simulink model "thermal_IGBT_Loss"  (R2024b)
settings: Solver=VariableStepAuto  StartTime=0.0  StopTime=10  RelTol=1e-3
values from neighbouring files (symbols this model uses):
  alpha_AS_dB_km = 0.40    (= 0.4)    [Inverter_new.m]    (also in init_pv_inverter.m = 0.26)
  alpha_S_dB_km = 0.20    (= 0.2)    [Inverter_new.m]    (also in init_pv_inverter.m = 0.24)
  f_sw = 2000    [blindval.m]    (also in init_pv_inverter.m)
  Pload = 2000    [blindval.m]    (also in init_pv_inverter.m)
  Rinterface_h = 0.02    [blindval.m]    (also in init_pv_inverter.m)
  Ron_IGBT = 1e-3    (= 0.001)    [blindval.m]    (also in init_pv_inverter.m)
  RTI = 90    [init_pv_inverter.m]
  T_ambient_fibre = Ta_K    (= 298.15)    [init_pv_inverter.m]
  Ta = test_cases(k,2)    [blindval.m]    (also in init_pv_inverter.m = 25)
  tf_IGBT = 63e-9    (= 6.3e-08)    [degradation_states.m]    (also in degradations_states_new.m; generate_degradation.m; init_pv_inverter.m; run_degradation.m)
  tr_IGBT = 11e-9    (= 1.1e-08)    [degradation_states.m]    (also in degradations_states_new.m; generate_degradation.m; init_pv_inverter.m; run_degradation.m)
  Ts_pwm = 5e-5    (= 5e-05)    [init_pv_inverter.m]
  Vdc = test_cases(k,3)    [blindval.m]    (also in init_pv_inverter.m = 600)
  Vf_IGBT = 0.8    [blindval.m]    (also in init_pv_inverter.m)
  x_fibre = 0:dx:L_fibre    [init_pv_inverter.m]
  x_fibre_km = x_fibre / 1000    [init_pv_inverter.m]
  x_inv_end = 7    [init_pv_inverter.m]
  x_inv_start = 5    [init_pv_inverter.m]
libraries: nesl_utility x13, ee_lib x8, fl_lib x6, simulink x6, eePwmGeneratorTwoLevel x1
settings Model: Creator=tf  LastModifiedBy=tf

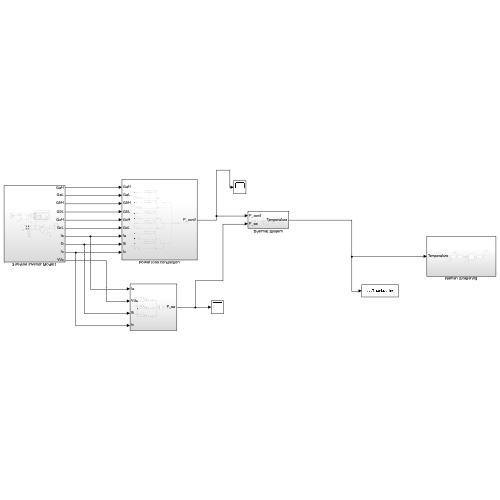
[thumbnail: Simulink's stored preview of the top-level diagram]
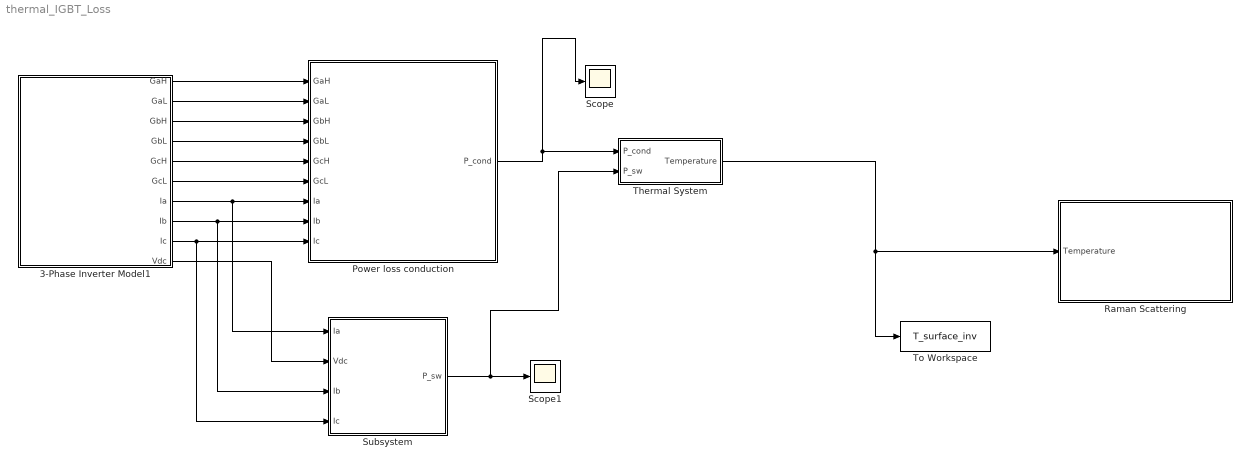
== system thermal_IGBT_Loss ==
  3-Phase Inverter Model1 : Subsystem
  Power loss conduction : Subsystem
  Raman Scattering : Subsystem
  Scope : Scope
  Scope1 : Scope
  Subsystem : Subsystem
  Thermal System : Subsystem
  To Workspace : ToWorkspace  VariableName=T_surface_inv  SaveFormat=Timeseries  SampleTime=0.01
  wires:
  Thermal System/1(Temperature) -> To Workspace/1, Raman Scattering/1(Temperature)
  3-Phase Inverter Model1/3(GbH) -> Power loss conduction/3(GbH)
  3-Phase Inverter Model1/7(Ia) -> Subsystem/1(Ia), Power loss conduction/7(Ia)
  3-Phase Inverter Model1/9(Ic) -> Subsystem/4(Ic), Power loss conduction/9(Ic)
  3-Phase Inverter Model1/2(GaL) -> Power loss conduction/2(GaL)
  3-Phase Inverter Model1/1(GaH) -> Power loss conduction/1(GaH)
  3-Phase Inverter Model1/5(GcH) -> Power loss conduction/5(GcH)
  3-Phase Inverter Model1/4(GbL) -> Power loss conduction/4(GbL)
  3-Phase Inverter Model1/6(GcL) -> Power loss conduction/6(GcL)
  3-Phase Inverter Model1/8(Ib) -> Subsystem/3(Ib), Power loss conduction/8(Ib)
  Power loss conduction/1(P_cond) -> Thermal System/1(P_cond), Scope/1
  3-Phase Inverter Model1/10(Vdc) -> Subsystem/2(Vdc)
  Subsystem/1(P_sw) -> Thermal System/2(P_sw), Scope1/1

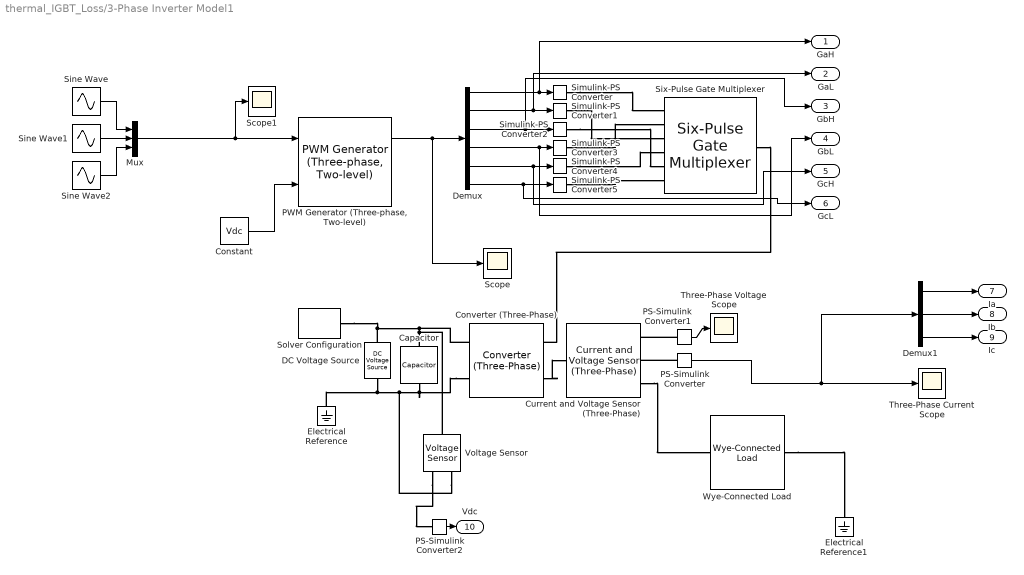
== system thermal_IGBT_Loss/3-Phase Inverter Model1 ==
  Capacitor : ee_lib/Passive/Capacitor  cap_option=ee.enum.passive.capacitor.capOption.const  c=1e-6 F  Cvec=[1e-05, 1e-06] F  Vvec=[0, 10] V  CV_table_symmetry=ee.enum.passive.capacitor.tableSymmetry.yes  f_vec=[1, 10] kHz  DFext_vec=[.8, 1.2]  enable_C_tol=ee.enum.toleranceApplication.none  averaging_period=0 s  C_tol=5  tol_distribution=ee.enum.toleranceDistribution.uniform  nSigma=4  r=0 Ohm  g=0 1/Ohm  enable_operating_limits=ee.enum.enable.no  operating_limit_action=ee.enum.passive.reportOpLim.warn  max_working_voltage_range=[-25, 25] V  power_rating=1 W  maxTemperature=85 degC  thermalEnable=false  thermalMass=1 J/K  fault_action=simscape.enum.assert.action.none  t_fault=1 s  i_specify=off  i_priority=None  i=0 A  i_nominal_specify=off  i_nominal_value=1  i_nominal_unit=A  v_specify=off  v_priority=High  v=600 V  v_nominal_specify=off  v_nominal_value=1  v_nominal_unit=V  vc_specify=on  vc_priority=High  vc=Vdc V  vc_nominal_specify=off  vc_nominal_value=1  vc_nominal_unit=V  T_specify=off  T_priority=None  T=298.15 K  T_nominal_specify=off  T_nominal_value=1  T_nominal_unit=K
  Constant : Constant  Value=Vdc
  Converter (Three-Phase) : ee_lib/Semiconductors & Converters/Converters/Converter (Three-Phase)  port_option=ee.enum.threePhasePort.composite  fidelity_option=ee.enum.converters.fidelity.equivalent_pwm  device_type=ee.enum.converters.switchingdevice.ideal  showThermalPort=true  K=0  Vth=6 V  Vgt=1 V  Vgt_off=-1 V  Ih=1 A  Vf=0.8 V  Ron=0.001 Ohm  Rds=0.001 Ohm  Goff=1e-6 1/Ohm  Eon_scalar=22.86e-3 J  Eoff_scalar=17.14e-3 J  Eoff_natural_commutation=10e-3 J  Voff=300 V  Iout_scalar=600 A  onCurrentMeasDelay=0 s  useCurrentFromPreviousCycle=false  useVoltageFromPreviousCycle=false  diode_param=ee.enum.converters.protectiondiode.nodynamics  diode_Vf=0.8 V  diode_Ron=0.001 Ohm  diode_Goff=1e-5 1/Ohm  diode_C=50 nF  diode_iRM=-235 A  diode_iF=300 A  diode_idot=-50 A/us  diode_trr_param=ee.enum.converters.diodetrr.trr_factor  diode_trr_factor=3  diode_trr=15 us  diode_Qrr=1500 s*uA  diode_rec_loss_model=ee.enum.diode.reverseRecoveryModel.fixed  diode_ErecVal=0 J  diode_scaleWithIandV=false  diode_ErecMat=zeros(2, 3) J  diode_TjrecVec=[298.15, 398.15] K  diode_IfrecVec=[.1, 1, 10] A  diode_IrecVal=10 A  diode_VrecVal=10 V  diode_tFilter=1 / 1000 / 100 s  thermal_network_parameterization=ee.enum.thermalNetworkTopology.external  Rth=[.08, .5] K/W  Rth_Cauer=[.08, .1, .5] K/W  Rth_Foster=[.08, .14, .22, .16] K/W  thermal_mass_parameterization=ee.enum.thermalNetwork.timeconstant  thermal_mass=[.01, .5] J/K  thermal_mass_Cauer=[.01, .1, .5] J/K  thermal_mass_Foster=[.001, .005, .05, .5] J/K  thermal_time_constant=[.001, .2] s  thermal_time_constant_Cauer=[.001, .1, .2] s  thermal_time_constant_Foster=[7e-05, .0007, .01, .08] s  thermal_mass_initial_temperatures=[25, 25] degC  thermal_mass_initial_temperatures_Cauer=[25, 25, 25] degC  junction_thermal_mass=0.01 J/K  Tvec_initial_Foster=[25, 25, 25, 25] degC  snubber_type=ee.enum.converters.snubber.exclude  Cs=1e-7 F  Rs=0.1 Ohm  Vce_loss=[0, 150, 300] V
  Current and Voltage Sensor (Three-Phase) : ee_lib/Sensors & Transducers/Current and Voltage Sensor (Three-Phase)  vMeasurementType=ee.enum.vmeasurement.lg  outputUnit=ee.enum.unit.si  SRated=100e6 A*V  VRated=24e3 V  I_specify=off  I_priority=None  I=[0, 0, 0] A  I_nominal_specify=off  I_nominal_value=1  I_nominal_unit=A  V_specify=off  V_priority=None  V=[0, 0, 0] V  V_nominal_specify=off  V_nominal_value=1  V_nominal_unit=V
      settings: InternalSimscapePortConfiguration="{\"Bottom\":[],\"Left\":[{\"id\":\"N1\",\"label\":\"~1\",\"type\":\"foundation.electrical.three_phase\"}],\"Right\":[{\"id\":\"V_output\",\"label\":\"V\",\"type\":\"output\"},{\"id\":\"I_output\",\"label\":\"I\",\"type\":\"output\"},{\"id\":\"N2\",\"label\":\"~2\",\"type\":\"foundation.electrical.three_phase\"}],\"Top\":[]}"
  DC Voltage Source : ee_lib/Additional Components/SPICE Sources/DC Voltage Source  DC=Vdc V
  Demux : Demux  Outputs=6
  Demux1 : Demux  Outputs=3
  Electrical Reference : fl_lib/Electrical/Electrical Elements/Electrical Reference
  Electrical Reference1 : fl_lib/Electrical/Electrical Elements/Electrical Reference
  Mux : Mux  Inputs=3
  PS-Simulink Converter : nesl_utility/PS-Simulink Converter  PhysicalDomain=network_engine_domain  SubClassName=ps_output  LeftPortType=input  RightPortType=output  PseudoPeriodic=off  Frequencies=[]  VectorFormat=inherit  Unit=A  AffineConversion=off
  PS-Simulink Converter1 : nesl_utility/PS-Simulink Converter  PhysicalDomain=network_engine_domain  SubClassName=ps_output  LeftPortType=input  RightPortType=output  PseudoPeriodic=off  Frequencies=[]  VectorFormat=inherit  Unit=V  AffineConversion=off
  PS-Simulink Converter2 : nesl_utility/PS-Simulink Converter  PhysicalDomain=network_engine_domain  SubClassName=ps_output  LeftPortType=input  RightPortType=output  PseudoPeriodic=off  Frequencies=[]  VectorFormat=inherit  Unit=V  AffineConversion=off
  "PWM Generator (Three-phase, Two-level)" : eePwmGeneratorTwoLevel/PWM Generator (Three-phase, Two-level)  PWMMode=Continuous PWM (CPWM)  CPWMMode=SPWM: sinusoidal PWM  DPWMMode=60 DPWM: 60 degree discontinuous PWM  fsw=f_sw  Ts=Ts_pwm
  Scope : Scope
  Scope1 : Scope
  Simulink-PS Converter{,1..5} (6 alike) : nesl_utility/Simulink-PS Converter  PhysicalDomain=network_engine_domain  SubClassName=ps_input  LeftPortType=input  RightPortType=output  PseudoPeriodic=off  Frequencies=[]  NoiseDistribution=none  NoiseParameters=[]  Unit=1  AffineConversion=off  FilteringAndDerivatives=provide  SimscapeFilterOrder=1  InputFilterTimeConstant=0.001  UdotUserProvided=0
  Sine Wave : Sin  Amplitude=0.8  Frequency=50  SampleTime=0
  Sine Wave1 : Sin  Amplitude=0.8  Frequency=50  Phase=-2*pi/3  SampleTime=0
  Sine Wave2 : Sin  Amplitude=0.8  Frequency=50  Phase=2*pi/3  SampleTime=0
  Six-Pulse Gate Multiplexer : ee_lib/Semiconductors & Converters/Converters/Six-Pulse Gate Multiplexer  port_option=ee.enum.controlport.ps
  Solver Configuration : nesl_utility/Solver Configuration  PhysicalDomain=network_engine_domain  SubClassName=solver  LeftPortType=input  RightPortType=generic  Tones=[]  Harmonics=[]  SimulateNoise=off  Profile=off  UseLocalSampling=off  EnableSwitchedLinearOptims=on  FrequencyDomain=off  UseCCode=off  RelTol=0.001  AbsTol=0.001  MinStep=1e-09  ToWorkspace=off  RevertToSquareIcSolve=off  NumHomotopyIterations=100  PhasorMode=off  PhasorModeNumHarmonics=1  ConsistencySolver=NEWTON_XTOL_AFTER_FTOL  IndexReductionMethod=DerivativeReplacement  DoDC=off  ResidualTolerance=1e-09  ConsistencyTolSource=GLOBAL  ConsistencyAbsTol=0.001  ConsistencyRelTol=0.001  ConsistencyTolFactor=0.001  UseLocalSolver=off  LocalSolverChoice=NE_BACKWARD_EULER_ADVANCER  ResolveIndetEquations=on  FunctionEvalNumThread=1  LocalSolverSampleTime=0.001  DoFixedCost=off  MaxNonlinIter=3  MaxModeIter=2  ComputeImpulses=off  ImpulseIterations=2  LinearAlgebra=auto  LinearAlgebraNumThread=0  EquationFormulation=NE_TIME_EF  DelaysMemoryBudget=1024  AutomaticFiltering=on  FilteringTimeConstant=0.001  PartitionStorageMethod=AS_NEEDED  PartitionMemoryBudget=1024  PartitionMethod=ROBUST  MultibodyUseLocalSolver=off  MultibodyLocalSolverChoice=ODE1  MultibodyLocalSolverSampleTime=0.001
  Three-Phase Current Scope : Scope
  Three-Phase Voltage Scope : Scope
  Voltage Sensor : fl_lib/Electrical/Electrical Sensors/Voltage Sensor
  Wye-Connected Load : ee_lib/Passive/RLC Assemblies/Wye-Connected Load  port_option=ee.enum.threePhasePort.composite  parameterization=ee.enum.rlc.parameterization.ratedpower  component_structure=ee.enum.rlc.structure.SeriesRL  component_structure_PQ=ee.enum.rlc.structure.SeriesRLC  R=1 Ohm  L=1e-3 H  C=1e-6 F  VRated=Vload_rated V  FRated=f_out Hz  P=Pload W  Qpos=Qind A*V  Qneg=Qcap A*V  R_parasitic=1e-6 Ohm  G_parasitic=1e-6 1/Ohm  R_parasitic_PQ=1e-6 Ohm  G_parasitic_PQ=1e-6 1/Ohm  Vmag0=24e3 V  Vang0=0 deg  Freq0=60 Hz  IL_specify=off  IL_priority=High  IL=[0, 0, 0] A  IL_nominal_specify=off  IL_nominal_value=1  IL_nominal_unit=A  VC_specify=off  VC_priority=High  VC=[0, 0, 0] V  VC_nominal_specify=off  VC_nominal_value=1  VC_nominal_unit=V
  GaH : Outport
  GaL : Outport  Port=2
  GbH : Outport  Port=3
  GbL : Outport  Port=4
  GcH : Outport  Port=5
  GcL : Outport  Port=6
  Ia : Outport  Port=7
  Ib : Outport  Port=8
  Ic : Outport  Port=9
  Vdc : Outport  Port=10
  wires:
  "PWM Generator (Three-phase, Two-level)"/1 -> Demux/1, Scope/1
  PS-Simulink Converter/1 -> Demux1/1, Three-Phase Current Scope/1
  Constant/1 -> "PWM Generator (Three-phase, Two-level)"/2
  Sine Wave/1 -> Mux/1
  Mux/1 -> Scope1/1, "PWM Generator (Three-phase, Two-level)"/1
  Demux/5 -> GcH/1, Simulink-PS Converter4/1
  Sine Wave1/1 -> Mux/2
  Demux/6 -> GcL/1, Simulink-PS Converter5/1
  Demux/4 -> GbL/1, Simulink-PS Converter3/1
  Demux/1 -> GaH/1, Simulink-PS Converter/1
  Sine Wave2/1 -> Mux/3
  Demux/2 -> GaL/1, Simulink-PS Converter1/1
  PS-Simulink Converter1/1 -> Three-Phase Voltage Scope/1
  Demux/3 -> GbH/1, Simulink-PS Converter2/1
  Demux1/1 -> Ia/1
  Demux1/2 -> Ib/1
  Demux1/3 -> Ic/1
  PS-Simulink Converter2/1 -> Vdc/1
  connections:
  Converter (Three-Phase)/RConn2 -- DC Voltage Source/RConn1 -- Electrical Reference/LConn1 -- Voltage Sensor/RConn2 -- Capacitor/RConn1
  Converter (Three-Phase)/RConn1 -- Voltage Sensor/LConn1 -- Capacitor/LConn1 -- DC Voltage Source/LConn1 -- Solver Configuration/RConn1
  Converter (Three-Phase)/LConn2 -- Current and Voltage Sensor (Three-Phase)/LConn1
  Six-Pulse Gate Multiplexer/RConn1 -- Converter (Three-Phase)/LConn1
  Simulink-PS Converter/RConn1 -- Six-Pulse Gate Multiplexer/LConn1
  PS-Simulink Converter/LConn1 -- Current and Voltage Sensor (Three-Phase)/RConn2
  Current and Voltage Sensor (Three-Phase)/RConn3 -- Wye-Connected Load/LConn1
  Wye-Connected Load/RConn1 -- Electrical Reference1/LConn1
  PS-Simulink Converter1/LConn1 -- Current and Voltage Sensor (Three-Phase)/RConn1
  Simulink-PS Converter3/RConn1 -- Six-Pulse Gate Multiplexer/LConn2
  Simulink-PS Converter1/RConn1 -- Six-Pulse Gate Multiplexer/LConn3
  Simulink-PS Converter4/RConn1 -- Six-Pulse Gate Multiplexer/LConn4
  Simulink-PS Converter2/RConn1 -- Six-Pulse Gate Multiplexer/LConn5
  Simulink-PS Converter5/RConn1 -- Six-Pulse Gate Multiplexer/LConn6
  Voltage Sensor/RConn1 -- PS-Simulink Converter2/LConn1

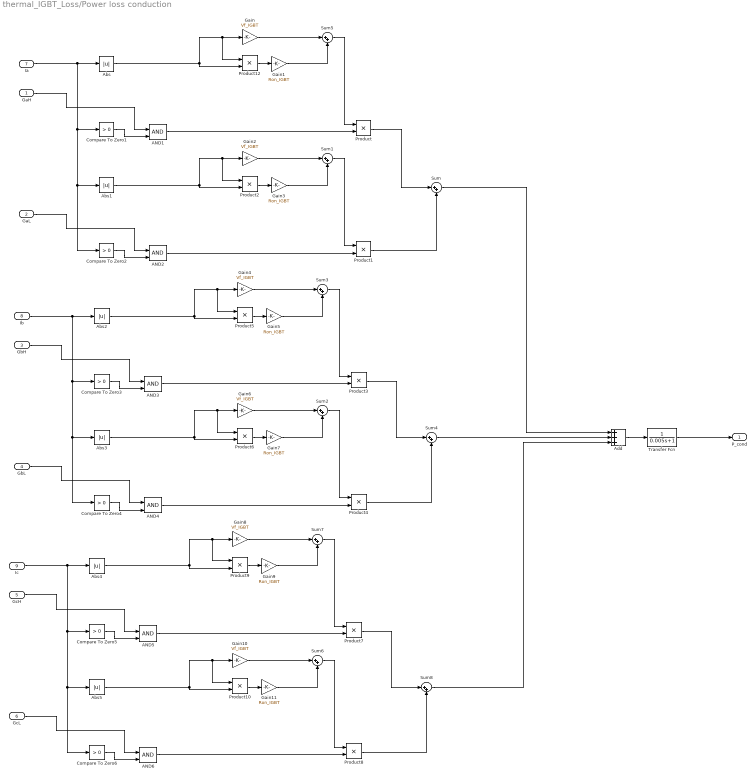
== system thermal_IGBT_Loss/Power loss conduction ==
  GaH : Inport
  GaL : Inport  Port=2
  GbH : Inport  Port=3
  GbL : Inport  Port=4
  GcH : Inport  Port=5
  GcL : Inport  Port=6
  Ia : Inport  Port=7
  Ib : Inport  Port=8
  Ic : Inport  Port=9
  AND{1..6} (6 alike) : Logic  IconShape=distinctive  AllPortsSameDT=off  OutDataTypeStr=boolean
  Abs{,1..5} (6 alike) : Abs  SaturateOnIntegerOverflow=off
  Add : Sum  Inputs=+++
  Compare To Zero{1..6} (6 alike) : simulink/Logic and Bit Operations/Compare To Zero  relop=>  OutDataTypeStr=boolean
  Gain{,2,4,6,8,10} (6 alike) : Gain  Gain=Vf_IGBT
  Gain{1,3,5,7,9,11} (6 alike) : Gain  Gain=Ron_IGBT
  Product{,1..10,12} (12 alike) : Product
  Sum{,1..8} (9 alike) : Sum  Inputs=|++
  Transfer Fcn : TransferFcn  Denominator=[0.005 1]
  P_cond : Outport
  wires:
  GaH/1 -> AND1/1
  Compare To Zero1/1 -> AND1/2
  Gain/1 -> Sum5/1
  Gain1/1 -> Sum5/2
  Product12/1 -> Gain1/1
  Abs/1 -> Product12/2, Product12/1, Gain/1
  AND1/1 -> Product/2
  Sum5/1 -> Product/1
  Product2/1 -> Gain3/1
  Ia/1 -> Compare To Zero2/1, Abs1/1, Compare To Zero1/1, Abs/1
  GaL/1 -> AND2/1
  Gain3/1 -> Sum1/2
  Abs1/1 -> Product2/2, Product2/1, Gain2/1
  AND2/1 -> Product1/2
  Gain2/1 -> Sum1/1
  Compare To Zero2/1 -> AND2/2
  Sum1/1 -> Product1/1
  AND4/1 -> Product4/2
  Gain5/1 -> Sum3/2
  Gain6/1 -> Sum2/1
  GbL/1 -> AND4/1
  Abs2/1 -> Product5/2, Product5/1, Gain4/1
  Abs3/1 -> Product6/2, Product6/1, Gain6/1
  Gain7/1 -> Sum2/2
  Product5/1 -> Gain5/1
  Compare To Zero4/1 -> AND4/2
  Product6/1 -> Gain7/1
  Sum2/1 -> Product4/1
  AND3/1 -> Product3/2
  GbH/1 -> AND3/1
  Gain4/1 -> Sum3/1
  Sum3/1 -> Product3/1
  Compare To Zero3/1 -> AND3/2
  Ib/1 -> Compare To Zero4/1, Abs3/1, Compare To Zero3/1, Abs2/1
  Product/1 -> Sum/1
  Product1/1 -> Sum/2
  Product3/1 -> Sum4/1
  Product4/1 -> Sum4/2
  Product10/1 -> Gain11/1
  Gain11/1 -> Sum6/2
  AND5/1 -> Product7/2
  Ic/1 -> Compare To Zero6/1, Abs5/1, Compare To Zero5/1, Abs4/1
  Abs5/1 -> Product10/2, Product10/1, Gain10/1
  Gain8/1 -> Sum7/1
  Product8/1 -> Sum8/2
  GcH/1 -> AND5/1
  Compare To Zero6/1 -> AND6/2
  Abs4/1 -> Product9/2, Product9/1, Gain8/1
  Sum6/1 -> Product8/1
  GcL/1 -> AND6/1
  Compare To Zero5/1 -> AND5/2
  Product9/1 -> Gain9/1
  Sum7/1 -> Product7/1
  Product7/1 -> Sum8/1
  AND6/1 -> Product8/2
  Gain9/1 -> Sum7/2
  Gain10/1 -> Sum6/1
  Sum/1 -> Add/1
  Sum4/1 -> Add/2
  Sum8/1 -> Add/3
  Add/1 -> Transfer Fcn/1
  Transfer Fcn/1 -> P_cond/1

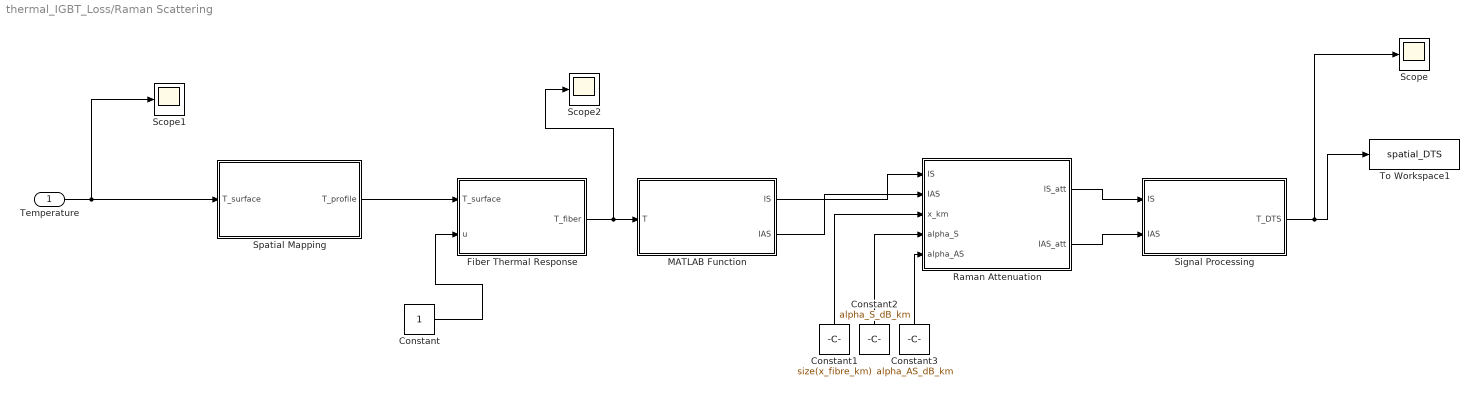
== system thermal_IGBT_Loss/Raman Scattering ==
  Temperature : Inport
  Constant : Constant
  Constant1 : Constant  Value=size(x_fibre_km)
  Constant2 : Constant  Value=alpha_S_dB_km
  Constant3 : Constant  Value=alpha_AS_dB_km
  Fiber Thermal Response : Subsystem
  MATLAB Function : MATLAB Function  TreatAsAtomicUnit=on
  Raman Attenuation : MATLAB Function  TreatAsAtomicUnit=on
  Scope : Scope
  Scope1 : Scope
  Scope2 : Scope
  Signal Processing : Subsystem
  Spatial Mapping : Subsystem
  To Workspace1 : ToWorkspace  VariableName=spatial_DTS  SaveFormat=Timeseries  SampleTime=0.01
  wires:
  Signal Processing/1(T_DTS) -> Scope/1, To Workspace1/1
  Fiber Thermal Response/1(T_fiber) -> Scope2/1, MATLAB Function/1(T)
  Constant/1 -> Fiber Thermal Response/2(u)
  Temperature/1 -> Scope1/1, Spatial Mapping/1(T_surface)
  Spatial Mapping/1(T_profile) -> Fiber Thermal Response/1(T_surface)
  Raman Attenuation/1(IS_att) -> Signal Processing/1(IS)
  Raman Attenuation/2(IAS_att) -> Signal Processing/2(IAS)
  MATLAB Function/1(IS) -> Raman Attenuation/1(IS)
  MATLAB Function/2(IAS) -> Raman Attenuation/2(IAS)
  Constant1/1 -> Raman Attenuation/3(x_km)
  Constant2/1 -> Raman Attenuation/4(alpha_S)
  Constant3/1 -> Raman Attenuation/5(alpha_AS)

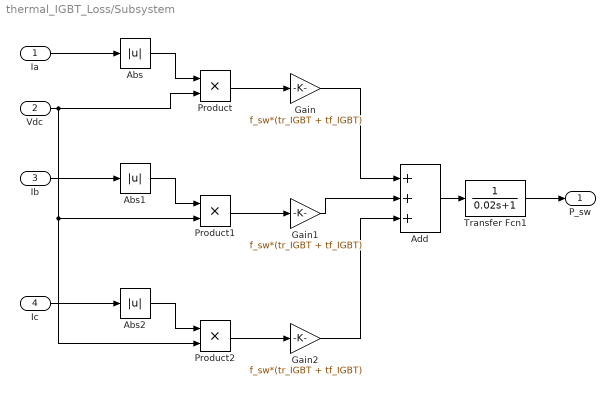
== system thermal_IGBT_Loss/Subsystem ==
  Ia : Inport
  Vdc : Inport  Port=2
  Ib : Inport  Port=3
  Ic : Inport  Port=4
  Abs : Abs  SaturateOnIntegerOverflow=off
  Abs1 : Abs  SaturateOnIntegerOverflow=off
  Abs2 : Abs  SaturateOnIntegerOverflow=off
  Add : Sum  Inputs=+++
  Gain : Gain  Gain=f_sw*(tr_IGBT + tf_IGBT)
  Gain1 : Gain  Gain=f_sw*(tr_IGBT + tf_IGBT)
  Gain2 : Gain  Gain=f_sw*(tr_IGBT + tf_IGBT)
  Product : Product
  Product1 : Product
  Product2 : Product
  Transfer Fcn1 : TransferFcn  Denominator=[0.02 1]
  P_sw : Outport
  wires:
  Ia/1 -> Abs/1
  Abs/1 -> Product/1
  Product/1 -> Gain/1
  Product1/1 -> Gain1/1
  Abs1/1 -> Product1/1
  Ib/1 -> Abs1/1
  Abs2/1 -> Product2/1
  Product2/1 -> Gain2/1
  Vdc/1 -> Product2/2, Product1/2, Product/2
  Ic/1 -> Abs2/1
  Add/1 -> Transfer Fcn1/1
  Gain/1 -> Add/1
  Gain1/1 -> Add/2
  Gain2/1 -> Add/3
  Transfer Fcn1/1 -> P_sw/1

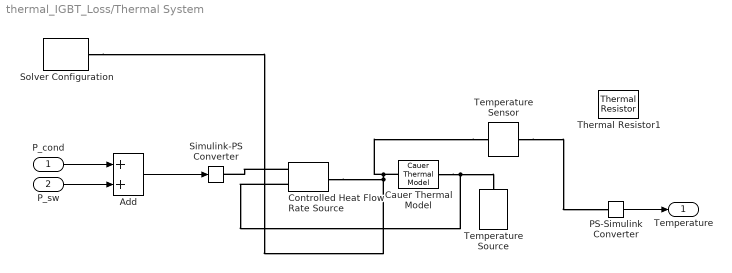
== system thermal_IGBT_Loss/Thermal System ==
  P_cond : Inport
  P_sw : Inport  Port=2
  Add : Sum
  Cauer Thermal Model : ee_lib/Passive/Thermal/Cauer Thermal Model  parameterize_foster=false  resistance_data=Rth K/W  tau_data=tau_th s  resistance_data_foster=[.0016, .0043, .0013, .0014] K/W  tau_data_foster=[.0068, .064, .32, 2] s  Tvec_specify=on  Tvec_priority=High  Tvec=Tinit K  Tvec_nominal_specify=off  Tvec_nominal_value=1  Tvec_nominal_unit=K  Q_A_specify=off  Q_A_priority=None  Q_A=0 W  Q_A_nominal_specify=off  Q_A_nominal_value=1  Q_A_nominal_unit=W  Q_B_specify=off  Q_B_priority=None  Q_B=0 W  Q_B_nominal_specify=off  Q_B_nominal_value=1  Q_B_nominal_unit=W
      settings: InternalSimscapePortConfiguration="{\"Bottom\":[],\"Left\":[{\"id\":\"A\",\"label\":\"A\",\"type\":\"foundation.thermal.thermal\"}],\"Right\":[{\"id\":\"B\",\"label\":\"B\",\"type\":\"foundation.thermal.thermal\"}],\"Top\":[]}"
  Controlled Heat Flow Rate Source : fl_lib/Thermal/Thermal Sources/Controlled Heat Flow Rate Source
  PS-Simulink Converter : nesl_utility/PS-Simulink Converter  PhysicalDomain=network_engine_domain  SubClassName=ps_output  LeftPortType=input  RightPortType=output  PseudoPeriodic=off  Frequencies=[]  VectorFormat=inherit  Unit=inherit  AffineConversion=off
  Simulink-PS Converter : nesl_utility/Simulink-PS Converter  PhysicalDomain=network_engine_domain  SubClassName=ps_input  LeftPortType=input  RightPortType=output  PseudoPeriodic=off  Frequencies=[]  NoiseDistribution=none  NoiseParameters=[]  Unit=W  AffineConversion=off  FilteringAndDerivatives=provide  SimscapeFilterOrder=1  InputFilterTimeConstant=0.001  UdotUserProvided=0
  Solver Configuration : nesl_utility/Solver Configuration  PhysicalDomain=network_engine_domain  SubClassName=solver  LeftPortType=input  RightPortType=generic  Tones=[]  Harmonics=[]  SimulateNoise=off  Profile=off  UseLocalSampling=off  EnableSwitchedLinearOptims=on  FrequencyDomain=off  UseCCode=off  RelTol=0.001  AbsTol=0.001  MinStep=1e-09  ToWorkspace=off  RevertToSquareIcSolve=off  NumHomotopyIterations=100  PhasorMode=off  PhasorModeNumHarmonics=1  ConsistencySolver=NEWTON_XTOL_AFTER_FTOL  IndexReductionMethod=DerivativeReplacement  DoDC=off  ResidualTolerance=1e-09  ConsistencyTolSource=GLOBAL  ConsistencyAbsTol=0.001  ConsistencyRelTol=0.001  ConsistencyTolFactor=0.001  UseLocalSolver=off  LocalSolverChoice=NE_BACKWARD_EULER_ADVANCER  ResolveIndetEquations=on  FunctionEvalNumThread=1  LocalSolverSampleTime=0.001  DoFixedCost=off  MaxNonlinIter=3  MaxModeIter=2  ComputeImpulses=off  ImpulseIterations=2  LinearAlgebra=auto  LinearAlgebraNumThread=0  EquationFormulation=NE_TIME_EF  DelaysMemoryBudget=1024  AutomaticFiltering=on  FilteringTimeConstant=0.001  PartitionStorageMethod=AS_NEEDED  PartitionMemoryBudget=1024  PartitionMethod=ROBUST  MultibodyUseLocalSolver=off  MultibodyLocalSolverChoice=ODE1  MultibodyLocalSolverSampleTime=0.001
  Temperature Sensor : fl_lib/Thermal/Thermal Sensors/Temperature Sensor  temperature_measure=foundation.enum.MeasurementReference.absolute
      settings: InternalSimscapePortConfiguration="{\"Bottom\":[],\"Left\":[{\"id\":\"A\",\"label\":\"A\",\"type\":\"foundation.thermal.thermal\"}],\"Right\":[{\"id\":\"T\",\"label\":\"T\",\"type\":\"output\"}],\"Top\":[]}"
  Temperature Source : fl_lib/Thermal/Thermal Sources/Temperature Source  temperature=Ta + 273.15 K
  Thermal Resistor1 : ee_lib/Passive/Thermal/Thermal Resistor  R=Rinterface_h K/W  T_specify=off  T_priority=None  T=0 K  T_nominal_specify=off  T_nominal_value=1  T_nominal_unit=K  Q_specify=off  Q_priority=None  Q=0 W  Q_nominal_specify=off  Q_nominal_value=1  Q_nominal_unit=W
      settings: InternalSimscapePortConfiguration="{\"Bottom\":[],\"Left\":[{\"id\":\"A\",\"label\":\"A\",\"type\":\"foundation.thermal.thermal\"}],\"Right\":[{\"id\":\"B\",\"label\":\"B\",\"type\":\"foundation.thermal.thermal\"}],\"Top\":[]}"
  Temperature : Outport
  wires:
  PS-Simulink Converter/1 -> Temperature/1
  P_cond/1 -> Add/1
  Add/1 -> Simulink-PS Converter/1
  P_sw/1 -> Add/2
  connections:
  Temperature Source/LConn1 -- Cauer Thermal Model/RConn1 -- Controlled Heat Flow Rate Source/RConn2
  Temperature Sensor/LConn1 -- Cauer Thermal Model/LConn1 -- Solver Configuration/RConn1 -- Controlled Heat Flow Rate Source/LConn1
  Temperature Sensor/RConn1 -- PS-Simulink Converter/LConn1
  Controlled Heat Flow Rate Source/RConn1 -- Simulink-PS Converter/RConn1

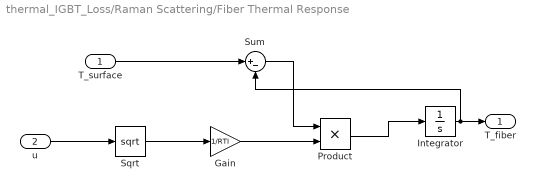
== system thermal_IGBT_Loss/Raman Scattering/Fiber Thermal Response ==
  T_surface : Inport
  u : Inport  Port=2
  Gain : Gain  Gain=1/RTI
  Integrator : Integrator  InitialCondition=298.15
  Product : Product
  Sqrt : Sqrt
  Sum : Sum  Inputs=|+-
  T_fiber : Outport
  wires:
  u/1 -> Sqrt/1
  Gain/1 -> Product/2
  Sqrt/1 -> Gain/1
  T_surface/1 -> Sum/1
  Integrator/1 -> Sum/2, T_fiber/1
  Sum/1 -> Product/1
  Product/1 -> Integrator/1

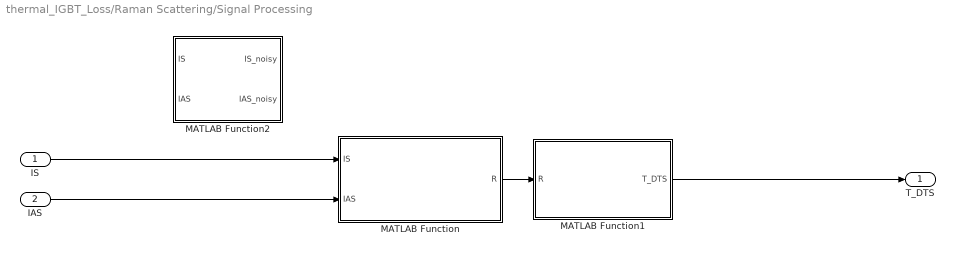
== system thermal_IGBT_Loss/Raman Scattering/Signal Processing ==
  IS : Inport
  IAS : Inport  Port=2
  MATLAB Function : MATLAB Function  TreatAsAtomicUnit=on
  MATLAB Function1 : MATLAB Function  TreatAsAtomicUnit=on
  MATLAB Function2 : MATLAB Function  TreatAsAtomicUnit=on
  T_DTS : Outport
  wires:
  MATLAB Function/1(R) -> MATLAB Function1/1(R)
  MATLAB Function1/1(T_DTS) -> T_DTS/1
  IS/1 -> MATLAB Function/1(IS)
  IAS/1 -> MATLAB Function/2(IAS)

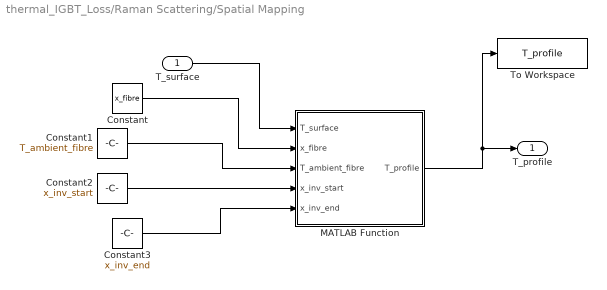
== system thermal_IGBT_Loss/Raman Scattering/Spatial Mapping ==
  T_surface : Inport
  Constant : Constant  Value=x_fibre
  Constant1 : Constant  Value=T_ambient_fibre
  Constant2 : Constant  Value=x_inv_start
  Constant3 : Constant  Value=x_inv_end
  MATLAB Function : MATLAB Function  TreatAsAtomicUnit=on
  To Workspace : ToWorkspace  VariableName=T_profile  SampleTime=-1
      settings: Decimation=200
  T_profile : Outport
  wires:
  T_surface/1 -> MATLAB Function/1(T_surface)
  MATLAB Function/1(T_profile) -> To Workspace/1, T_profile/1
  Constant/1 -> MATLAB Function/2(x_fibre)
  Constant1/1 -> MATLAB Function/3(T_ambient_fibre)
  Constant2/1 -> MATLAB Function/4(x_inv_start)
  Constant3/1 -> MATLAB Function/5(x_inv_end)

== matlab function thermal_IGBT_Loss/Raman Scattering/MATLAB Function ==
  data: T input; IS output; IAS output
function [IS, IAS] = RamanScattering(T)
%#codegen

N = 41;

IS  = zeros(1,N);
IAS = zeros(1,N);

h  = 6.62607015e-34;
c  = 299792458;
kB = 1.380649e-23;

ramanShift_cm = 440;
ramanShift_m  = ramanShift_cm * 100;

thetaR = h*c*ramanShift_m/kB;

T_safe = max(T,1);

nPh = 1 ./ (exp(thetaR ./ T_safe) - 1);

IS  = nPh + 1;
IAS = nPh;

end

== matlab function thermal_IGBT_Loss/Raman Scattering/Spatial Mapping/MATLAB Function ==
  data: T_surface input; T_profile output; x_fibre input; T_ambient_fibre input; x_inv_start input; x_inv_end input
function T_profile = spatial_mapping(T_surface, x_fibre, ...
    T_ambient_fibre, x_inv_start, x_inv_end)
%#codegen

N = 41;

% Fixed-size output
T_profile = T_ambient_fibre .* ones(1,N);

% Inverter sensing region
idx = (x_fibre >= x_inv_start) & ...
      (x_fibre <= x_inv_end);

% Apply inverter surface temperature
T_profile(idx) = T_surface;

end

== matlab function thermal_IGBT_Loss/Raman Scattering/Signal Processing/MATLAB Function ==
  data: IS input; R output; IAS input
function R = RamanRatio(IS, IAS)
%#codegen


%Safeguard to prevent division by zero
IS = max(IS,1e-12);


R = IAS./IS;

end

== matlab function thermal_IGBT_Loss/Raman Scattering/Signal Processing/MATLAB Function1 ==
  data: R input; T_DTS output
function T_DTS = Reconstruct_Temperature(R)

%#codegen

%constants
h = 6.62607015 * 10^-34; % Plancks Constant
c = 299792458; % Speed of light
kB = 1.380649 * 10^-23; % Boltzmann Constant

% Raman shift for silica
raman_shift_cm = 440;                   % [cm^-1]
raman_shift_m  = raman_shift_cm * 100;  % [m^-1]

% Prevent invalid logarithm values
R_safe = min(max(R, 1e-12), 1 - 1e-12);

% Temperature reconstruction
T_DTS = -(h*c*raman_shift_m) ./ (kB*log(R_safe));

end

== matlab function thermal_IGBT_Loss/Raman Scattering/Raman Attenuation ==
  data: IS input; IS_att output; IAS input; x_km input; alpha_S input; alpha_AS input; IAS_att output
function [IS_att, IAS_att] = RamanAttenuation( ...
    IS, IAS, x_km, alpha_S, alpha_AS)
%#codegen

% Wavelength-dependent attenuation
loss_S  = 10.^(-(alpha_S  .* x_km) ./ 10);
loss_AS = 10.^(-(alpha_AS .* x_km) ./ 10);

IS_att  = IS  .* loss_S;
IAS_att = IAS .* loss_AS;

end

== matlab function thermal_IGBT_Loss/Raman Scattering/Signal Processing/MATLAB Function2 ==
  settings: updateMethod=DISCRETE  sampleTime=0.01
  data: IS input; IS_noisy output; IAS input; IAS_noisy output
function [IS_noisy, IAS_noisy] = RamanNoise(IS, IAS)
%#codegen

SNR_dB = 15;
SNR_linear = 10^(SNR_dB/10);

% Stokes noise
Ps_S = mean(IS.^2);
Pn_S = Ps_S ./ SNR_linear;
sigma_S = sqrt(Pn_S);

% Anti-Stokes noise
Ps_AS = mean(IAS.^2);
Pn_AS = Ps_AS ./ SNR_linear;
sigma_AS = sqrt(Pn_AS);

% Independent Gaussian noise 
IS_noisy  = IS  + sigma_S  .* randn(size(IS));
IAS_noisy = IAS + sigma_AS .* randn(size(IAS));

end
